simulink model "PowerFlow_SUSAN"  (R2022b)
settings: Solver=FixedStepAuto  StartTime=0.0  StopTime=10  FixedStep=0.02  RelTol=1e-3
libraries: Lib_EMTAT x193
(part 1 of 3)
settings Model: Creator=sbianco1  LastModifiedBy=sbianco1
settings SolverCC: AlgebraicLoopSolver=TrustRegion
settings DebuggingCC: UnconnectedInputMsg=warning  UnconnectedOutputMsg=warning  UnconnectedLineMsg=warning  SFMachineParentedDataDiag=warning
settings ModelReferenceCC: EnableRefExpFcnMdlSchedulingChecks=on
settings RTWCC: DLArmComputeVersion=19.05

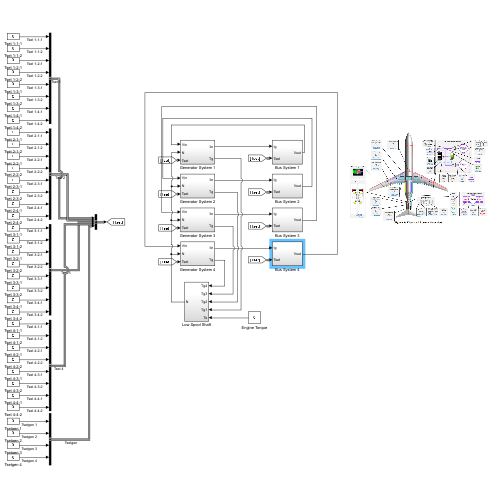
[thumbnail: Simulink's stored preview of the top-level diagram]
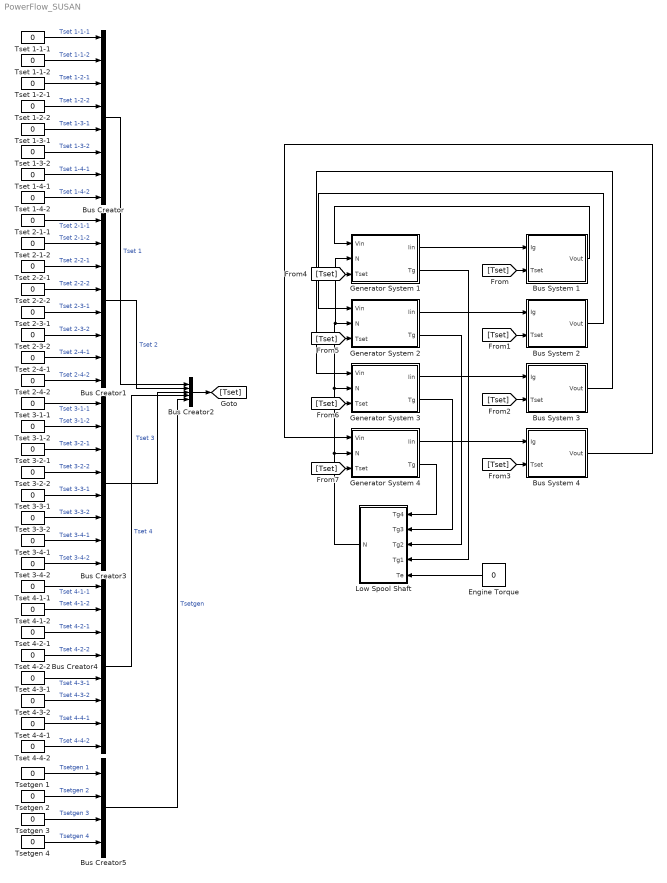
== system PowerFlow_SUSAN ==
  Bus Creator{,1,3..4} (4 alike) : BusCreator  Inputs=8
  Bus Creator2 : BusCreator  Inputs=5
  Bus Creator5 : BusCreator  Inputs=4
  Bus System 1 : Subsystem
  Bus System 2 : Subsystem
  Bus System 3 : Subsystem
  Bus System 4 : Subsystem
  Engine Torque : Constant  Value=0
  Generator System 1 : Subsystem
  Generator System 2 : Subsystem
  Generator System 3 : Subsystem
  Generator System 4 : Subsystem
  Low Spool Shaft : Subsystem
  Tset 1-1-1 : Constant  Value=0
  Tset 1-1-2 : Constant  Value=0
  Tset 1-2-1 : Constant  Value=0
  Tset 1-2-2 : Constant  Value=0
  Tset 1-3-1 : Constant  Value=0
  Tset 1-3-2 : Constant  Value=0
  Tset 1-4-1 : Constant  Value=0
  Tset 1-4-2 : Constant  Value=0
  Tset 2-1-1 : Constant  Value=0
  Tset 2-1-2 : Constant  Value=0
  Tset 2-2-1 : Constant  Value=0
  Tset 2-2-2 : Constant  Value=0
  Tset 2-3-1 : Constant  Value=0
  Tset 2-3-2 : Constant  Value=0
  Tset 2-4-1 : Constant  Value=0
  Tset 2-4-2 : Constant  Value=0
  Tset 3-1-1 : Constant  Value=0
  Tset 3-1-2 : Constant  Value=0
  Tset 3-2-1 : Constant  Value=0
  Tset 3-2-2 : Constant  Value=0
  Tset 3-3-1 : Constant  Value=0
  Tset 3-3-2 : Constant  Value=0
  Tset 3-4-1 : Constant  Value=0
  Tset 3-4-2 : Constant  Value=0
  Tset 4-1-1 : Constant  Value=0
  Tset 4-1-2 : Constant  Value=0
  Tset 4-2-1 : Constant  Value=0
  Tset 4-2-2 : Constant  Value=0
  Tset 4-3-1 : Constant  Value=0
  Tset 4-3-2 : Constant  Value=0
  Tset 4-4-1 : Constant  Value=0
  Tset 4-4-2 : Constant  Value=0
  Tsetgen {1..4} (4 alike) : Constant  Value=0
  wires:
  Engine Torque/1 -> Low Spool Shaft/5(Te)
  Generator System 1/2(Tg) -> Low Spool Shaft/4(Tg1)
  Generator System 2/2(Tg) -> Low Spool Shaft/3(Tg2)
  Generator System 3/2(Tg) -> Low Spool Shaft/2(Tg3)
  Generator System 4/2(Tg) -> Low Spool Shaft/1(Tg4)
  Low Spool Shaft/1(N) -> Generator System 4/2(N), Generator System 3/2(N), Generator System 2/2(N), Generator System 1/2(N)
  Generator System 1/1(Iin) -> Bus System 1/1(Ig)
  Bus System 1/1(Vout) -> Generator System 1/1(Vin)
  Generator System 2/1(Iin) -> Bus System 2/1(Ig)
  Generator System 3/1(Iin) -> Bus System 3/1(Ig)
  Generator System 4/1(Iin) -> Bus System 4/1(Ig)
  Bus System 2/1(Vout) -> Generator System 2/1(Vin)
  Bus System 3/1(Vout) -> Generator System 3/1(Vin)
  Bus System 4/1(Vout) -> Generator System 4/1(Vin)
  Tset 1-4-2/1 -> Bus Creator/8  "Tset 1-4-2"
  Tset 1-4-1/1 -> Bus Creator/7  "Tset 1-4-1"
  Tset 1-3-2/1 -> Bus Creator/6  "Tset 1-3-2"
  Tset 1-3-1/1 -> Bus Creator/5  "Tset 1-3-1"
  Tset 1-2-2/1 -> Bus Creator/4  "Tset 1-2-2"
  Tset 1-2-1/1 -> Bus Creator/3  "Tset 1-2-1"
  Tset 1-1-2/1 -> Bus Creator/2  "Tset 1-1-2"
  Tset 1-1-1/1 -> Bus Creator/1  "Tset 1-1-1"
  Bus Creator/1 -> Bus Creator2/1  "Tset 1"
  Bus Creator1/1 -> Bus Creator2/2  "Tset 2"
  Tset 2-1-1/1 -> Bus Creator1/1  "Tset 2-1-1"
  Tset 2-1-2/1 -> Bus Creator1/2  "Tset 2-1-2"
  Tset 2-2-1/1 -> Bus Creator1/3  "Tset 2-2-1"
  Tset 2-2-2/1 -> Bus Creator1/4  "Tset 2-2-2"
  Tset 2-3-1/1 -> Bus Creator1/5  "Tset 2-3-1"
  Tset 2-3-2/1 -> Bus Creator1/6  "Tset 2-3-2"
  Tset 2-4-1/1 -> Bus Creator1/7  "Tset 2-4-1"
  Tset 2-4-2/1 -> Bus Creator1/8  "Tset 2-4-2"
  Bus Creator2/1 -> [Tset]
  [Tset] -> Bus System 1/2(Tset)
  [Tset] -> Bus System 2/2(Tset)
  [Tset] -> Bus System 3/2(Tset)
  [Tset] -> Bus System 4/2(Tset)
  Tset 3-4-2/1 -> Bus Creator3/8  "Tset 3-4-2"
  Tset 3-4-1/1 -> Bus Creator3/7  "Tset 3-4-1"
  Tset 3-3-2/1 -> Bus Creator3/6  "Tset 3-3-2"
  Tset 3-3-1/1 -> Bus Creator3/5  "Tset 3-3-1"
  Tset 3-2-2/1 -> Bus Creator3/4  "Tset 3-2-2"
  Tset 3-2-1/1 -> Bus Creator3/3  "Tset 3-2-1"
  Tset 3-1-2/1 -> Bus Creator3/2  "Tset 3-1-2"
  Tset 3-1-1/1 -> Bus Creator3/1  "Tset 3-1-1"
  Bus Creator3/1 -> Bus Creator2/3  "Tset 3"
  Bus Creator4/1 -> Bus Creator2/4  "Tset 4"
  Tset 4-1-1/1 -> Bus Creator4/1  "Tset 4-1-1"
  Tset 4-1-2/1 -> Bus Creator4/2  "Tset 4-1-2"
  Tset 4-2-1/1 -> Bus Creator4/3  "Tset 4-2-1"
  Tset 4-2-2/1 -> Bus Creator4/4  "Tset 4-2-2"
  Tset 4-3-1/1 -> Bus Creator4/5  "Tset 4-3-1"
  Tset 4-3-2/1 -> Bus Creator4/6  "Tset 4-3-2"
  Tset 4-4-1/1 -> Bus Creator4/7  "Tset 4-4-1"
  Tset 4-4-2/1 -> Bus Creator4/8  "Tset 4-4-2"
  Tsetgen 1/1 -> Bus Creator5/1  "Tsetgen 1"
  Tsetgen 2/1 -> Bus Creator5/2  "Tsetgen 2"
  Tsetgen 3/1 -> Bus Creator5/3  "Tsetgen 3"
  Tsetgen 4/1 -> Bus Creator5/4  "Tsetgen 4"
  Bus Creator5/1 -> Bus Creator2/5  "Tsetgen"
  [Tset] -> Generator System 1/3(Tset)
  [Tset] -> Generator System 2/3(Tset)
  [Tset] -> Generator System 3/3(Tset)
  [Tset] -> Generator System 4/3(Tset)

== system PowerFlow_SUSAN/Bus System 1 ==
  Ig : Inport
  Tset : Inport  Port=2
  Bus Selector : BusSelector  OutputSignals=Tset 1.Tset 1-1-1,Tset 1.Tset 1-1-2  OutputAsBus=on
  Bus Selector1 : BusSelector  OutputSignals=Tset 1.Tset 1-2-1,Tset 1.Tset 1-2-2  OutputAsBus=on
  Bus Selector2 : BusSelector  OutputSignals=Tset 1.Tset 1-3-1,Tset 1.Tset 1-3-2  OutputAsBus=on
  Bus Selector3 : BusSelector  OutputSignals=Tset 1.Tset 1-4-1,Tset 1.Tset 1-4-2  OutputAsBus=on
  Current Distribution1 : Lib_EMTAT/Components/Power Flow/Current Distribution
      settings: SourceProductName=EMTAT
  Demux : Demux
  Mux : Mux
  Propulsor System 1 : Subsystem
  Propulsor System 2 : Subsystem
  Propulsor System 3 : Subsystem
  Propulsor System 4 : Subsystem
  Terminator : Terminator
  Terminator1 : Terminator
  Terminator2 : Terminator
  Vout : Outport
  wires:
  Propulsor System 3/2(Idmd) -> Mux/3
  Demux/1 -> Propulsor System 1/1(Iin)
  Demux/3 -> Propulsor System 3/1(Iin)
  Demux/4 -> Propulsor System 4/1(Iin)
  Propulsor System 3/1(Vout) -> Terminator1/1
  Propulsor System 2/2(Idmd) -> Mux/2
  Demux/2 -> Propulsor System 2/1(Iin)
  Propulsor System 4/1(Vout) -> Terminator2/1
  Propulsor System 2/1(Vout) -> Terminator/1
  Propulsor System 4/2(Idmd) -> Mux/4
  Propulsor System 1/2(Idmd) -> Mux/1
  Propulsor System 1/1(Vout) -> Vout/1
  Ig/1 -> Current Distribution1/1
  Tset/1 -> Bus Selector1/1, Bus Selector2/1, Bus Selector3/1, Bus Selector/1
  [Tset_1] -> Propulsor System 1/2(Tset)
  [Tset_2] -> Propulsor System 2/2(Tset)
  [Tset_3] -> Propulsor System 3/2(Tset)
  [Tset_4] -> Propulsor System 4/2(Tset)
  Bus Selector/1 -> [Tset_1]
  Bus Selector1/1 -> [Tset_2]
  Bus Selector2/1 -> [Tset_3]
  Bus Selector3/1 -> [Tset_4]
  Mux/1 -> Current Distribution1/2
  Current Distribution1/1 -> Demux/1

== system PowerFlow_SUSAN/Bus System 2 ==
  Ig : Inport
  Tset : Inport  Port=2
  Bus Selector : BusSelector  OutputSignals=Tset 2.Tset 2-1-1,Tset 2.Tset 2-1-2  OutputAsBus=on
  Bus Selector1 : BusSelector  OutputSignals=Tset 2.Tset 2-2-1,Tset 2.Tset 2-2-2  OutputAsBus=on
  Bus Selector2 : BusSelector  OutputSignals=Tset 2.Tset 2-3-1,Tset 2.Tset 2-3-2  OutputAsBus=on
  Bus Selector3 : BusSelector  OutputSignals=Tset 2.Tset 2-4-1,Tset 2.Tset 2-4-2  OutputAsBus=on
  Current Distribution1 : Lib_EMTAT/Components/Power Flow/Current Distribution
      settings: SourceProductName=EMTAT
  Demux : Demux
  Mux : Mux
  Propulsor System 1 : Subsystem
  Propulsor System 2 : Subsystem
  Propulsor System 3 : Subsystem
  Propulsor System 4 : Subsystem
  Terminator : Terminator
  Terminator1 : Terminator
  Terminator2 : Terminator
  Vout : Outport
  wires:
  Current Distribution1/1 -> Demux/1
  Mux/1 -> Current Distribution1/2
  Bus Selector3/1 -> [Tset_4]
  Bus Selector2/1 -> [Tset_3]
  Bus Selector1/1 -> [Tset_2]
  Bus Selector/1 -> [Tset_1]
  [Tset_4] -> Propulsor System 4/2(Tset)
  [Tset_3] -> Propulsor System 3/2(Tset)
  [Tset_2] -> Propulsor System 2/2(Tset)
  [Tset_1] -> Propulsor System 1/2(Tset)
  Tset/1 -> Bus Selector/1, Bus Selector3/1, Bus Selector2/1, Bus Selector1/1
  Ig/1 -> Current Distribution1/1
  Propulsor System 1/1(Vout) -> Vout/1
  Propulsor System 1/2(Idmd) -> Mux/1
  Propulsor System 4/2(Idmd) -> Mux/4
  Propulsor System 2/1(Vout) -> Terminator/1
  Propulsor System 4/1(Vout) -> Terminator2/1
  Demux/2 -> Propulsor System 2/1(Iin)
  Propulsor System 2/2(Idmd) -> Mux/2
  Propulsor System 3/1(Vout) -> Terminator1/1
  Demux/4 -> Propulsor System 4/1(Iin)
  Demux/3 -> Propulsor System 3/1(Iin)
  Demux/1 -> Propulsor System 1/1(Iin)
  Propulsor System 3/2(Idmd) -> Mux/3

== system PowerFlow_SUSAN/Bus System 3 ==
  Ig : Inport
  Tset : Inport  Port=2
  Bus Selector : BusSelector  OutputSignals=Tset 3.Tset 3-1-1,Tset 3.Tset 3-1-2  OutputAsBus=on
  Bus Selector1 : BusSelector  OutputSignals=Tset 3.Tset 3-2-1,Tset 3.Tset 3-2-2  OutputAsBus=on
  Bus Selector2 : BusSelector  OutputSignals=Tset 3.Tset 3-3-1,Tset 3.Tset 3-3-2  OutputAsBus=on
  Bus Selector3 : BusSelector  OutputSignals=Tset 3.Tset 3-4-1,Tset 3.Tset 3-4-2  OutputAsBus=on
  Current Distribution1 : Lib_EMTAT/Components/Power Flow/Current Distribution
      settings: SourceProductName=EMTAT
  Demux : Demux
  Mux : Mux
  Propulsor System 1 : Subsystem
  Propulsor System 2 : Subsystem
  Propulsor System 3 : Subsystem
  Propulsor System 4 : Subsystem
  Terminator : Terminator
  Terminator1 : Terminator
  Terminator2 : Terminator
  Vout : Outport
  wires:
  Propulsor System 3/2(Idmd) -> Mux/3
  Demux/1 -> Propulsor System 1/1(Iin)
  Demux/3 -> Propulsor System 3/1(Iin)
  Demux/4 -> Propulsor System 4/1(Iin)
  Propulsor System 3/1(Vout) -> Terminator1/1
  Propulsor System 2/2(Idmd) -> Mux/2
  Demux/2 -> Propulsor System 2/1(Iin)
  Propulsor System 4/1(Vout) -> Terminator2/1
  Propulsor System 2/1(Vout) -> Terminator/1
  Propulsor System 4/2(Idmd) -> Mux/4
  Propulsor System 1/2(Idmd) -> Mux/1
  Propulsor System 1/1(Vout) -> Vout/1
  Ig/1 -> Current Distribution1/1
  Tset/1 -> Bus Selector1/1, Bus Selector2/1, Bus Selector3/1, Bus Selector/1
  [Tset_1] -> Propulsor System 1/2(Tset)
  [Tset_2] -> Propulsor System 2/2(Tset)
  [Tset_3] -> Propulsor System 3/2(Tset)
  [Tset_4] -> Propulsor System 4/2(Tset)
  Bus Selector/1 -> [Tset_1]
  Bus Selector1/1 -> [Tset_2]
  Bus Selector2/1 -> [Tset_3]
  Bus Selector3/1 -> [Tset_4]
  Mux/1 -> Current Distribution1/2
  Current Distribution1/1 -> Demux/1

== system PowerFlow_SUSAN/Bus System 4 ==
  Ig : Inport
  Tset : Inport  Port=2
  Bus Selector : BusSelector  OutputSignals=Tset 4.Tset 4-1-1,Tset 4.Tset 4-1-2  OutputAsBus=on
  Bus Selector1 : BusSelector  OutputSignals=Tset 4.Tset 4-2-1,Tset 4.Tset 4-2-2  OutputAsBus=on
  Bus Selector2 : BusSelector  OutputSignals=Tset 4.Tset 4-3-1,Tset 4.Tset 4-3-2  OutputAsBus=on
  Bus Selector3 : BusSelector  OutputSignals=Tset 4.Tset 4-4-1,Tset 4.Tset 4-4-2  OutputAsBus=on
  Current Distribution1 : Lib_EMTAT/Components/Power Flow/Current Distribution
      settings: SourceProductName=EMTAT
  Demux : Demux
  Mux : Mux
  Propulsor System 1 : Subsystem
  Propulsor System 2 : Subsystem
  Propulsor System 3 : Subsystem
  Propulsor System 4 : Subsystem
  Terminator : Terminator
  Terminator1 : Terminator
  Terminator2 : Terminator
  Vout : Outport
  wires:
  Current Distribution1/1 -> Demux/1
  Mux/1 -> Current Distribution1/2
  Bus Selector3/1 -> [Tset_4]
  Bus Selector2/1 -> [Tset_3]
  Bus Selector1/1 -> [Tset_2]
  Bus Selector/1 -> [Tset_1]
  [Tset_4] -> Propulsor System 4/2(Tset)
  [Tset_3] -> Propulsor System 3/2(Tset)
  [Tset_2] -> Propulsor System 2/2(Tset)
  [Tset_1] -> Propulsor System 1/2(Tset)
  Tset/1 -> Bus Selector/1, Bus Selector3/1, Bus Selector2/1, Bus Selector1/1
  Ig/1 -> Current Distribution1/1
  Propulsor System 1/1(Vout) -> Vout/1
  Propulsor System 1/2(Idmd) -> Mux/1
  Propulsor System 4/2(Idmd) -> Mux/4
  Propulsor System 2/1(Vout) -> Terminator/1
  Propulsor System 4/1(Vout) -> Terminator2/1
  Demux/2 -> Propulsor System 2/1(Iin)
  Propulsor System 2/2(Idmd) -> Mux/2
  Propulsor System 3/1(Vout) -> Terminator1/1
  Demux/4 -> Propulsor System 4/1(Iin)
  Demux/3 -> Propulsor System 3/1(Iin)
  Demux/1 -> Propulsor System 1/1(Iin)
  Propulsor System 3/2(Idmd) -> Mux/3

== system PowerFlow_SUSAN/Generator System 1 ==
  Vin : Inport
  N : Inport  Port=2
  Tset : Inport  Port=3
  Bus Selector : BusSelector  OutputSignals=Tsetgen.Tsetgen 1
  Cable2 : Lib_EMTAT/Components/Power Flow/Cable  R=0.2
      settings: SourceProductName=EMTAT
  Constant{,1..4} (5 alike) : Constant  Value=0
  Inverter/Rectifier (Sink) : Lib_EMTAT/Components/Power Flow/DC-AC Inverter  X_C_VoltageInVec_M=[0 400]  Y_C_RMSCurrentOutVec_M=[0 300]  T_C_PowLossArray_M=[1000 1000; 1000 1000]  K_e=0.0503  FM=0  Plosslim=0
      settings: SourceProductName=EMTAT
  Motor/Generator (Sink)2 : Lib_EMTAT/Components/Power Flow/Three Phase Electric Machine (Sink)  X_C_SpeedVec_M=[0 100 1000 5000]  Y_C_TorqueVec_M=[0 10 100 150]  T_C_EffArray_M=0.99*ones(4,4)  FM=0
      settings: SourceProductName=EMTAT
  Terminator{1,9..10,14..16} (6 alike) : Terminator
  Unit Delay : UnitDelay  SampleTime=-1  HasFrameUpgradeWarning=on
  Iin : Outport
  Tg : Outport  Port=2
  wires:
  Unit Delay/1 -> Cable2/4
  Inverter/Rectifier (Sink)/2 -> Terminator15/1
  Motor/Generator (Sink)2/4 -> Inverter/Rectifier (Sink)/3
  Inverter/Rectifier (Sink)/4 -> Cable2/2
  Cable2/1 -> Inverter/Rectifier (Sink)/1
  Motor/Generator (Sink)2/1 -> Tg/1
  Tset/1 -> Bus Selector/1
  Cable2/5 -> Unit Delay/1
  [N_G] -> Inverter/Rectifier (Sink)/2
  Motor/Generator (Sink)2/2 -> Terminator16/1
  Inverter/Rectifier (Sink)/3 -> Terminator14/1
  Cable2/3 -> Terminator10/1
  Inverter/Rectifier (Sink)/1 -> Motor/Generator (Sink)2/1
  [N_G] -> Motor/Generator (Sink)2/2
  Cable2/2 -> Terminator9/1
  Vin/1 -> Cable2/1
  Cable2/4 -> Iin/1
  N/1 -> [N_G]
  Bus Selector/1 -> Motor/Generator (Sink)2/3  "<Tsetgen 1>"
  Constant/1 -> Inverter/Rectifier (Sink)/4
  Constant1/1 -> Cable2/3
  Constant2/1 -> Inverter/Rectifier (Sink)/5
  Constant3/1 -> Motor/Generator (Sink)2/4
  Constant4/1 -> Motor/Generator (Sink)2/5
  Motor/Generator (Sink)2/3 -> Terminator1/1

== system PowerFlow_SUSAN/Generator System 2 ==
  Vin : Inport
  N : Inport  Port=2
  Tset : Inport  Port=3
  Bus Selector : BusSelector  OutputSignals=Tsetgen.Tsetgen 1
  Cable2 : Lib_EMTAT/Components/Power Flow/Cable  R=0.2
      settings: SourceProductName=EMTAT
  Constant{,1..4} (5 alike) : Constant  Value=0
  Inverter/Rectifier (Sink) : Lib_EMTAT/Components/Power Flow/DC-AC Inverter  X_C_VoltageInVec_M=[0 400]  Y_C_RMSCurrentOutVec_M=[0 300]  T_C_PowLossArray_M=[1000 1000; 1000 1000]  K_e=0.0503  FM=0  Plosslim=0
      settings: SourceProductName=EMTAT
  Motor/Generator (Sink)2 : Lib_EMTAT/Components/Power Flow/Three Phase Electric Machine (Sink)  X_C_SpeedVec_M=[0 100 1000 5000]  Y_C_TorqueVec_M=[0 10 100 150]  T_C_EffArray_M=0.99*ones(4,4)  FM=0
      settings: SourceProductName=EMTAT
  Terminator{1,9..10,14..16} (6 alike) : Terminator
  Unit Delay : UnitDelay  SampleTime=-1  HasFrameUpgradeWarning=on
  Iin : Outport
  Tg : Outport  Port=2
  wires:
  Motor/Generator (Sink)2/3 -> Terminator1/1
  Constant4/1 -> Motor/Generator (Sink)2/5
  Constant3/1 -> Motor/Generator (Sink)2/4
  Constant2/1 -> Inverter/Rectifier (Sink)/5
  Constant1/1 -> Cable2/3
  Constant/1 -> Inverter/Rectifier (Sink)/4
  Bus Selector/1 -> Motor/Generator (Sink)2/3  "<Tsetgen 1>"
  N/1 -> [N_G]
  Cable2/4 -> Iin/1
  Vin/1 -> Cable2/1
  Cable2/2 -> Terminator9/1
  [N_G] -> Motor/Generator (Sink)2/2
  Inverter/Rectifier (Sink)/1 -> Motor/Generator (Sink)2/1
  Cable2/3 -> Terminator10/1
  Inverter/Rectifier (Sink)/3 -> Terminator14/1
  Motor/Generator (Sink)2/2 -> Terminator16/1
  [N_G] -> Inverter/Rectifier (Sink)/2
  Cable2/5 -> Unit Delay/1
  Tset/1 -> Bus Selector/1
  Motor/Generator (Sink)2/1 -> Tg/1
  Cable2/1 -> Inverter/Rectifier (Sink)/1
  Inverter/Rectifier (Sink)/4 -> Cable2/2
  Motor/Generator (Sink)2/4 -> Inverter/Rectifier (Sink)/3
  Inverter/Rectifier (Sink)/2 -> Terminator15/1
  Unit Delay/1 -> Cable2/4

== system PowerFlow_SUSAN/Generator System 3 ==
  Vin : Inport
  N : Inport  Port=2
  Tset : Inport  Port=3
  Bus Selector : BusSelector  OutputSignals=Tsetgen.Tsetgen 1
  Cable2 : Lib_EMTAT/Components/Power Flow/Cable  R=0.2
      settings: SourceProductName=EMTAT
  Constant{,1..4} (5 alike) : Constant  Value=0
  Inverter/Rectifier (Sink) : Lib_EMTAT/Components/Power Flow/DC-AC Inverter  X_C_VoltageInVec_M=[0 400]  Y_C_RMSCurrentOutVec_M=[0 300]  T_C_PowLossArray_M=[1000 1000; 1000 1000]  K_e=0.0503  FM=0  Plosslim=0
      settings: SourceProductName=EMTAT
  Motor/Generator (Sink)2 : Lib_EMTAT/Components/Power Flow/Three Phase Electric Machine (Sink)  X_C_SpeedVec_M=[0 100 1000 5000]  Y_C_TorqueVec_M=[0 10 100 150]  T_C_EffArray_M=0.99*ones(4,4)  FM=0
      settings: SourceProductName=EMTAT
  Terminator{1,9..10,14..16} (6 alike) : Terminator
  Unit Delay : UnitDelay  SampleTime=-1  HasFrameUpgradeWarning=on
  Iin : Outport
  Tg : Outport  Port=2
  wires:
  Unit Delay/1 -> Cable2/4
  Inverter/Rectifier (Sink)/2 -> Terminator15/1
  Motor/Generator (Sink)2/4 -> Inverter/Rectifier (Sink)/3
  Inverter/Rectifier (Sink)/4 -> Cable2/2
  Cable2/1 -> Inverter/Rectifier (Sink)/1
  Motor/Generator (Sink)2/1 -> Tg/1
  Tset/1 -> Bus Selector/1
  Cable2/5 -> Unit Delay/1
  [N_G] -> Inverter/Rectifier (Sink)/2
  Motor/Generator (Sink)2/2 -> Terminator16/1
  Inverter/Rectifier (Sink)/3 -> Terminator14/1
  Cable2/3 -> Terminator10/1
  Inverter/Rectifier (Sink)/1 -> Motor/Generator (Sink)2/1
  [N_G] -> Motor/Generator (Sink)2/2
  Cable2/2 -> Terminator9/1
  Vin/1 -> Cable2/1
  Cable2/4 -> Iin/1
  N/1 -> [N_G]
  Bus Selector/1 -> Motor/Generator (Sink)2/3  "<Tsetgen 1>"
  Constant/1 -> Inverter/Rectifier (Sink)/4
  Constant1/1 -> Cable2/3
  Constant2/1 -> Inverter/Rectifier (Sink)/5
  Constant3/1 -> Motor/Generator (Sink)2/4
  Constant4/1 -> Motor/Generator (Sink)2/5
  Motor/Generator (Sink)2/3 -> Terminator1/1

== system PowerFlow_SUSAN/Generator System 4 ==
  Vin : Inport
  N : Inport  Port=2
  Tset : Inport  Port=3
  Bus Selector : BusSelector  OutputSignals=Tsetgen.Tsetgen 1
  Cable2 : Lib_EMTAT/Components/Power Flow/Cable  R=0.2
      settings: SourceProductName=EMTAT
  Constant{,1..4} (5 alike) : Constant  Value=0
  Inverter/Rectifier (Sink) : Lib_EMTAT/Components/Power Flow/DC-AC Inverter  X_C_VoltageInVec_M=[0 400]  Y_C_RMSCurrentOutVec_M=[0 300]  T_C_PowLossArray_M=[1000 1000; 1000 1000]  K_e=0.0503  FM=0  Plosslim=0
      settings: SourceProductName=EMTAT
  Motor/Generator (Sink)2 : Lib_EMTAT/Components/Power Flow/Three Phase Electric Machine (Sink)  X_C_SpeedVec_M=[0 100 1000 5000]  Y_C_TorqueVec_M=[0 10 100 150]  T_C_EffArray_M=0.99*ones(4,4)  FM=0
      settings: SourceProductName=EMTAT
  Terminator{1,9..10,14..16} (6 alike) : Terminator
  Unit Delay : UnitDelay  SampleTime=-1  HasFrameUpgradeWarning=on
  Iin : Outport
  Tg : Outport  Port=2
  wires:
  Motor/Generator (Sink)2/3 -> Terminator1/1
  Constant4/1 -> Motor/Generator (Sink)2/5
  Constant3/1 -> Motor/Generator (Sink)2/4
  Constant2/1 -> Inverter/Rectifier (Sink)/5
  Constant1/1 -> Cable2/3
  Constant/1 -> Inverter/Rectifier (Sink)/4
  Bus Selector/1 -> Motor/Generator (Sink)2/3  "<Tsetgen 1>"
  N/1 -> [N_G]
  Cable2/4 -> Iin/1
  Vin/1 -> Cable2/1
  Cable2/2 -> Terminator9/1
  [N_G] -> Motor/Generator (Sink)2/2
  Inverter/Rectifier (Sink)/1 -> Motor/Generator (Sink)2/1
  Cable2/3 -> Terminator10/1
  Inverter/Rectifier (Sink)/3 -> Terminator14/1
  Motor/Generator (Sink)2/2 -> Terminator16/1
  [N_G] -> Inverter/Rectifier (Sink)/2
  Cable2/5 -> Unit Delay/1
  Tset/1 -> Bus Selector/1
  Motor/Generator (Sink)2/1 -> Tg/1
  Cable2/1 -> Inverter/Rectifier (Sink)/1
  Inverter/Rectifier (Sink)/4 -> Cable2/2
  Motor/Generator (Sink)2/4 -> Inverter/Rectifier (Sink)/3
  Inverter/Rectifier (Sink)/2 -> Terminator15/1
  Unit Delay/1 -> Cable2/4

== system PowerFlow_SUSAN/Low Spool Shaft ==
  Tg4 : Inport
  Tg3 : Inport  Port=2
  Tg2 : Inport  Port=3
  Tg1 : Inport  Port=4
  Te : Inport  Port=5
  Constant : Constant  Value=0
  Integrator : Integrator  InitialCondition=5000
  Mechanical Shaft3 : Lib_EMTAT/Components/Power Flow/Mechanical Shaft  J=0.01  B=0.001
      settings: SourceProductName=EMTAT
  Mux1 : Mux  Inputs=5
  Terminator5 : Terminator
  Terminator7 : Terminator
  N : Outport
  wires:
  Mux1/1 -> Mechanical Shaft3/1
  Integrator/1 -> Mechanical Shaft3/3, N/1
  Tg1/1 -> Mux1/1
  Tg4/1 -> Mux1/4
  Tg3/1 -> Mux1/3
  Tg2/1 -> Mux1/2
  Te/1 -> Mux1/5
  Mechanical Shaft3/1 -> Terminator5/1
  Mechanical Shaft3/2 -> Terminator7/1
  Mechanical Shaft3/3 -> Integrator/1
  Constant/1 -> Mechanical Shaft3/2

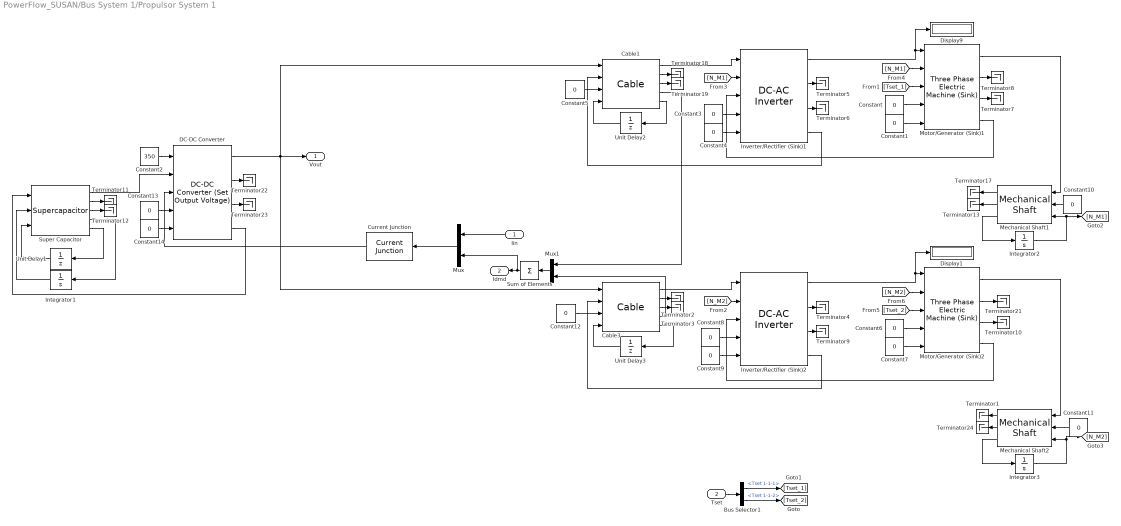
== system PowerFlow_SUSAN/Bus System 1/Propulsor System 1 ==
  Iin : Inport
  Tset : Inport  Port=2
  Bus Selector1 : BusSelector  OutputSignals=Tset 1-1-1,Tset 1-1-2
  Cable1 : Lib_EMTAT/Components/Power Flow/Cable  R=0.2
      settings: SourceProductName=EMTAT
  Cable3 : Lib_EMTAT/Components/Power Flow/Cable  R=0.2
      settings: SourceProductName=EMTAT
  Constant{,1,3..14} (14 alike) : Constant  Value=0
  Constant2 : Constant  Value=350
  Current Junction : Lib_EMTAT/Components/Power Flow/Current Junction  Nb=1
      settings: SourceProductName=EMTAT
      settings: AttributesFormatString=|
      | Current Junction
      | Version: %<LibraryVersion>
  DC-DC Converter : Lib_EMTAT/Components/Power Flow/DC-DC Converter (Set Output Voltage)  X_Vin_VoltageVec_M=[0 100 1000 5000]  Y_Iout_CurrentVec_M=[0 10 100 150]  T_C_PlossArray_M=0.98*ones(4,4)  FM=0  Plosslim=0
      settings: SourceProductName=EMTAT
  Display1 : Display
  Display9 : Display
  Integrator1 : Integrator  InitialCondition=150
  Integrator2 : Integrator  InitialCondition=2000
  Integrator3 : Integrator  InitialCondition=2000
  Inverter/Rectifier (Sink)1 : Lib_EMTAT/Components/Power Flow/DC-AC Inverter  X_C_VoltageInVec_M=[0 400]  Y_C_RMSCurrentOutVec_M=[0 300]  T_C_PowLossArray_M=[1000 1000;1000 1000]  K_e=0.0503  FM=0  Plosslim=0
      settings: SourceProductName=EMTAT
  Inverter/Rectifier (Sink)2 : Lib_EMTAT/Components/Power Flow/DC-AC Inverter  X_C_VoltageInVec_M=[0 400]  Y_C_RMSCurrentOutVec_M=[0 300]  T_C_PowLossArray_M=[1000 1000;1000 1000]  K_e=0.0503  FM=0  Plosslim=0
      settings: SourceProductName=EMTAT
  Mechanical Shaft1 : Lib_EMTAT/Components/Power Flow/Mechanical Shaft  J=0.01  B=0.001
      settings: SourceProductName=EMTAT
  Mechanical Shaft2 : Lib_EMTAT/Components/Power Flow/Mechanical Shaft  J=0.01  B=0.001
      settings: SourceProductName=EMTAT
  Motor/Generator (Sink)1 : Lib_EMTAT/Components/Power Flow/Three Phase Electric Machine (Sink)  X_C_SpeedVec_M=[0 100 1000 5000]  Y_C_TorqueVec_M=[0 10 100 150]  T_C_EffArray_M=0.99*ones(4,4)  FM=0
      settings: SourceProductName=EMTAT
  Motor/Generator (Sink)2 : Lib_EMTAT/Components/Power Flow/Three Phase Electric Machine (Sink)  X_C_SpeedVec_M=[0 100 1000 5000]  Y_C_TorqueVec_M=[0 10 100 150]  T_C_EffArray_M=0.99*ones(4,4)  FM=0
      settings: SourceProductName=EMTAT
  Mux : Mux  Inputs=2
  Mux1 : Mux  Inputs=2
  Sum of Elements : Sum  Inputs=+
  Super Capacitor : Lib_EMTAT/Components/Power Flow/Supercapacitor  C=130  ESR=0.02  TSE=0  BlkNm=double(gcb)
      settings: SourceProductName=EMTAT
  Terminator{1..13,17..19,21..24} (20 alike) : Terminator
  Unit Delay1 : UnitDelay  SampleTime=-1  HasFrameUpgradeWarning=on
  Unit Delay2 : UnitDelay  SampleTime=-1  HasFrameUpgradeWarning=on
  Unit Delay3 : UnitDelay  SampleTime=-1  HasFrameUpgradeWarning=on
  Vout : Outport
  Idmd : Outport  Port=2
  wires:
  Iin/1 -> Mux/1
  Mechanical Shaft2/3 -> Integrator3/1
  [Tset_1] -> Motor/Generator (Sink)1/3
  DC-DC Converter/1 -> Cable3/1, Vout/1, Cable1/1
  Motor/Generator (Sink)1/4 -> Inverter/Rectifier (Sink)1/3
  Super Capacitor/4 -> Integrator1/1
  Super Capacitor/1 -> DC-DC Converter/2
  [N_M1] -> Motor/Generator (Sink)1/2
  Mechanical Shaft1/2 -> Terminator13/1
  Unit Delay2/1 -> Cable1/4
  Cable3/2 -> Terminator2/1
  DC-DC Converter/4 -> Super Capacitor/1
  Current Junction/1 -> DC-DC Converter/3
  Mux/1 -> Current Junction/1
  Integrator2/1 -> [N_M1], Mechanical Shaft1/3
  Cable1/1 -> Inverter/Rectifier (Sink)1/1
  [N_M1] -> Inverter/Rectifier (Sink)1/2
  Cable3/5 -> Unit Delay3/1
  Inverter/Rectifier (Sink)1/1 -> Motor/Generator (Sink)1/1, Display9/1
  Super Capacitor/2 -> Terminator11/1
  Cable3/4 -> Mux1/2
  Integrator3/1 -> [N_M2], Mechanical Shaft2/3
  Cable1/3 -> Terminator19/1
  Unit Delay3/1 -> Cable3/4
  Inverter/Rectifier (Sink)1/4 -> Cable1/2
  Integrator1/1 -> Super Capacitor/2
  Cable1/5 -> Unit Delay2/1
  Inverter/Rectifier (Sink)1/3 -> Terminator6/1
  Super Capacitor/5 -> Unit Delay1/1
  Unit Delay1/1 -> Super Capacitor/3
  Cable1/4 -> Mux1/1
  Constant2/1 -> DC-DC Converter/1
  Motor/Generator (Sink)1/2 -> Terminator8/1
  Cable3/3 -> Terminator3/1
  Motor/Generator (Sink)2/1 -> Mechanical Shaft2/1
  Cable1/2 -> Terminator18/1
  Super Capacitor/3 -> Terminator12/1
  Motor/Generator (Sink)2/2 -> Terminator21/1
  Mechanical Shaft1/1 -> Terminator17/1
  DC-DC Converter/2 -> Terminator22/1
  DC-DC Converter/3 -> Terminator23/1
  Inverter/Rectifier (Sink)1/2 -> Terminator5/1
  Motor/Generator (Sink)1/1 -> Mechanical Shaft1/1
  Mux1/1 -> Sum of Elements/1
  Sum of Elements/1 -> Mux/2, Idmd/1
  Bus Selector1/1 -> [Tset_1]  "<Tset 1-1-1>"
  Bus Selector1/2 -> [Tset_2]  "<Tset 1-1-2>"
  Tset/1 -> Bus Selector1/1
  Constant/1 -> Motor/Generator (Sink)1/4
  Constant1/1 -> Motor/Generator (Sink)1/5
  Motor/Generator (Sink)1/3 -> Terminator7/1
  Constant3/1 -> Inverter/Rectifier (Sink)1/4
  Constant4/1 -> Inverter/Rectifier (Sink)1/5
  Constant5/1 -> Cable1/3
  Constant9/1 -> Inverter/Rectifier (Sink)2/5
  Inverter/Rectifier (Sink)2/2 -> Terminator4/1
  Constant7/1 -> Motor/Generator (Sink)2/5
  [N_M2] -> Inverter/Rectifier (Sink)2/2
  Inverter/Rectifier (Sink)2/3 -> Terminator9/1
  [Tset_2] -> Motor/Generator (Sink)2/3
  Inverter/Rectifier (Sink)2/4 -> Cable3/2
  Constant6/1 -> Motor/Generator (Sink)2/4
  Motor/Generator (Sink)2/4 -> Inverter/Rectifier (Sink)2/3
  Cable3/1 -> Inverter/Rectifier (Sink)2/1
  [N_M2] -> Motor/Generator (Sink)2/2
  Inverter/Rectifier (Sink)2/1 -> Motor/Generator (Sink)2/1, Display1/1
  Constant8/1 -> Inverter/Rectifier (Sink)2/4
  Motor/Generator (Sink)2/3 -> Terminator10/1
  Mechanical Shaft1/3 -> Integrator2/1
  Constant10/1 -> Mechanical Shaft1/2
  Constant11/1 -> Mechanical Shaft2/2
  Mechanical Shaft2/1 -> Terminator1/1
  Mechanical Shaft2/2 -> Terminator24/1
  Constant12/1 -> Cable3/3
  Constant13/1 -> DC-DC Converter/4
  Constant14/1 -> DC-DC Converter/5

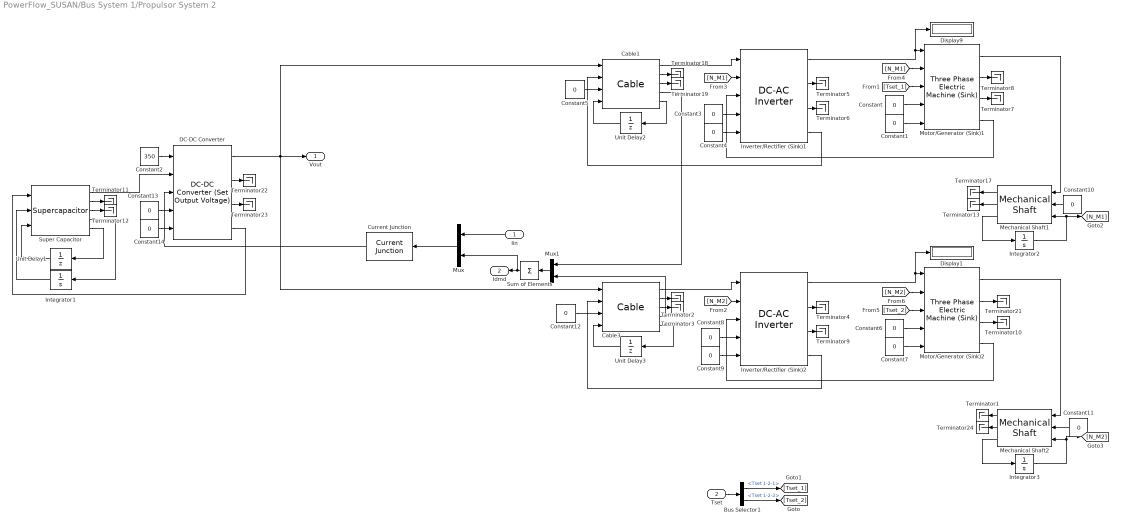
== system PowerFlow_SUSAN/Bus System 1/Propulsor System 2 ==
  Iin : Inport
  Tset : Inport  Port=2
  Bus Selector1 : BusSelector  OutputSignals=Tset 1-2-1,Tset 1-2-2
  Cable1 : Lib_EMTAT/Components/Power Flow/Cable  R=0.2
      settings: SourceProductName=EMTAT
  Cable3 : Lib_EMTAT/Components/Power Flow/Cable  R=0.2
      settings: SourceProductName=EMTAT
  Constant{,1,3..14} (14 alike) : Constant  Value=0
  Constant2 : Constant  Value=350
  Current Junction : Lib_EMTAT/Components/Power Flow/Current Junction  Nb=1
      settings: SourceProductName=EMTAT
      settings: AttributesFormatString=|
      | Current Junction
      | Version: %<LibraryVersion>
  DC-DC Converter : Lib_EMTAT/Components/Power Flow/DC-DC Converter (Set Output Voltage)  X_Vin_VoltageVec_M=[0 100 1000 5000]  Y_Iout_CurrentVec_M=[0 10 100 150]  T_C_PlossArray_M=0.98*ones(4,4)  FM=0  Plosslim=0
      settings: SourceProductName=EMTAT
  Display1 : Display
  Display9 : Display
  Integrator1 : Integrator  InitialCondition=150
  Integrator2 : Integrator  InitialCondition=2000
  Integrator3 : Integrator  InitialCondition=2000
  Inverter/Rectifier (Sink)1 : Lib_EMTAT/Components/Power Flow/DC-AC Inverter  X_C_VoltageInVec_M=[0 400]  Y_C_RMSCurrentOutVec_M=[0 300]  T_C_PowLossArray_M=[1000 1000;1000 1000]  K_e=0.0503  FM=0  Plosslim=0
      settings: SourceProductName=EMTAT
  Inverter/Rectifier (Sink)2 : Lib_EMTAT/Components/Power Flow/DC-AC Inverter  X_C_VoltageInVec_M=[0 400]  Y_C_RMSCurrentOutVec_M=[0 300]  T_C_PowLossArray_M=[1000 1000;1000 1000]  K_e=0.0503  FM=0  Plosslim=0
      settings: SourceProductName=EMTAT
  Mechanical Shaft1 : Lib_EMTAT/Components/Power Flow/Mechanical Shaft  J=0.01  B=0.001
      settings: SourceProductName=EMTAT
  Mechanical Shaft2 : Lib_EMTAT/Components/Power Flow/Mechanical Shaft  J=0.01  B=0.001
      settings: SourceProductName=EMTAT
  Motor/Generator (Sink)1 : Lib_EMTAT/Components/Power Flow/Three Phase Electric Machine (Sink)  X_C_SpeedVec_M=[0 100 1000 5000]  Y_C_TorqueVec_M=[0 10 100 150]  T_C_EffArray_M=0.99*ones(4,4)  FM=0
      settings: SourceProductName=EMTAT
  Motor/Generator (Sink)2 : Lib_EMTAT/Components/Power Flow/Three Phase Electric Machine (Sink)  X_C_SpeedVec_M=[0 100 1000 5000]  Y_C_TorqueVec_M=[0 10 100 150]  T_C_EffArray_M=0.99*ones(4,4)  FM=0
      settings: SourceProductName=EMTAT
  Mux : Mux  Inputs=2
  Mux1 : Mux  Inputs=2
  Sum of Elements : Sum  Inputs=+
  Super Capacitor : Lib_EMTAT/Components/Power Flow/Supercapacitor  C=130  ESR=0.02  TSE=0  BlkNm=double(gcb)
      settings: SourceProductName=EMTAT
  Terminator{1..13,17..19,21..24} (20 alike) : Terminator
  Unit Delay1 : UnitDelay  SampleTime=-1  HasFrameUpgradeWarning=on
  Unit Delay2 : UnitDelay  SampleTime=-1  HasFrameUpgradeWarning=on
  Unit Delay3 : UnitDelay  SampleTime=-1  HasFrameUpgradeWarning=on
  Vout : Outport
  Idmd : Outport  Port=2
  wires:
  Constant14/1 -> DC-DC Converter/5
  Constant13/1 -> DC-DC Converter/4
  Constant12/1 -> Cable3/3
  Mechanical Shaft2/2 -> Terminator24/1
  Mechanical Shaft2/1 -> Terminator1/1
  Constant11/1 -> Mechanical Shaft2/2
  Constant10/1 -> Mechanical Shaft1/2
  Mechanical Shaft1/3 -> Integrator2/1
  Motor/Generator (Sink)2/3 -> Terminator10/1
  Constant8/1 -> Inverter/Rectifier (Sink)2/4
  Inverter/Rectifier (Sink)2/1 -> Display1/1, Motor/Generator (Sink)2/1
  [N_M2] -> Motor/Generator (Sink)2/2
  Cable3/1 -> Inverter/Rectifier (Sink)2/1
  Motor/Generator (Sink)2/4 -> Inverter/Rectifier (Sink)2/3
  Constant6/1 -> Motor/Generator (Sink)2/4
  Inverter/Rectifier (Sink)2/4 -> Cable3/2
  [Tset_2] -> Motor/Generator (Sink)2/3
  Inverter/Rectifier (Sink)2/3 -> Terminator9/1
  [N_M2] -> Inverter/Rectifier (Sink)2/2
  Constant7/1 -> Motor/Generator (Sink)2/5
  Inverter/Rectifier (Sink)2/2 -> Terminator4/1
  Constant9/1 -> Inverter/Rectifier (Sink)2/5
  Constant5/1 -> Cable1/3
  Constant4/1 -> Inverter/Rectifier (Sink)1/5
  Constant3/1 -> Inverter/Rectifier (Sink)1/4
  Motor/Generator (Sink)1/3 -> Terminator7/1
  Constant1/1 -> Motor/Generator (Sink)1/5
  Constant/1 -> Motor/Generator (Sink)1/4
  Tset/1 -> Bus Selector1/1
  Bus Selector1/2 -> [Tset_2]  "<Tset 1-2-2>"
  Bus Selector1/1 -> [Tset_1]  "<Tset 1-2-1>"
  Sum of Elements/1 -> Idmd/1, Mux/2
  Mux1/1 -> Sum of Elements/1
  Motor/Generator (Sink)1/1 -> Mechanical Shaft1/1
  Inverter/Rectifier (Sink)1/2 -> Terminator5/1
  DC-DC Converter/3 -> Terminator23/1
  DC-DC Converter/2 -> Terminator22/1
  Mechanical Shaft1/1 -> Terminator17/1
  Motor/Generator (Sink)2/2 -> Terminator21/1
  Super Capacitor/3 -> Terminator12/1
  Cable1/2 -> Terminator18/1
  Motor/Generator (Sink)2/1 -> Mechanical Shaft2/1
  Cable3/3 -> Terminator3/1
  Motor/Generator (Sink)1/2 -> Terminator8/1
  Constant2/1 -> DC-DC Converter/1
  Cable1/4 -> Mux1/1
  Unit Delay1/1 -> Super Capacitor/3
  Super Capacitor/5 -> Unit Delay1/1
  Inverter/Rectifier (Sink)1/3 -> Terminator6/1
  Cable1/5 -> Unit Delay2/1
  Integrator1/1 -> Super Capacitor/2
  Inverter/Rectifier (Sink)1/4 -> Cable1/2
  Unit Delay3/1 -> Cable3/4
  Cable1/3 -> Terminator19/1
  Integrator3/1 -> Mechanical Shaft2/3, [N_M2]
  Cable3/4 -> Mux1/2
  Super Capacitor/2 -> Terminator11/1
  Inverter/Rectifier (Sink)1/1 -> Display9/1, Motor/Generator (Sink)1/1
  Cable3/5 -> Unit Delay3/1
  [N_M1] -> Inverter/Rectifier (Sink)1/2
  Cable1/1 -> Inverter/Rectifier (Sink)1/1
  Integrator2/1 -> Mechanical Shaft1/3, [N_M1]
  Mux/1 -> Current Junction/1
  Current Junction/1 -> DC-DC Converter/3
  DC-DC Converter/4 -> Super Capacitor/1
  Cable3/2 -> Terminator2/1
  Unit Delay2/1 -> Cable1/4
  Mechanical Shaft1/2 -> Terminator13/1
  [N_M1] -> Motor/Generator (Sink)1/2
  Super Capacitor/1 -> DC-DC Converter/2
  Super Capacitor/4 -> Integrator1/1
  Motor/Generator (Sink)1/4 -> Inverter/Rectifier (Sink)1/3
  DC-DC Converter/1 -> Cable1/1, Vout/1, Cable3/1
  [Tset_1] -> Motor/Generator (Sink)1/3
  Mechanical Shaft2/3 -> Integrator3/1
  Iin/1 -> Mux/1

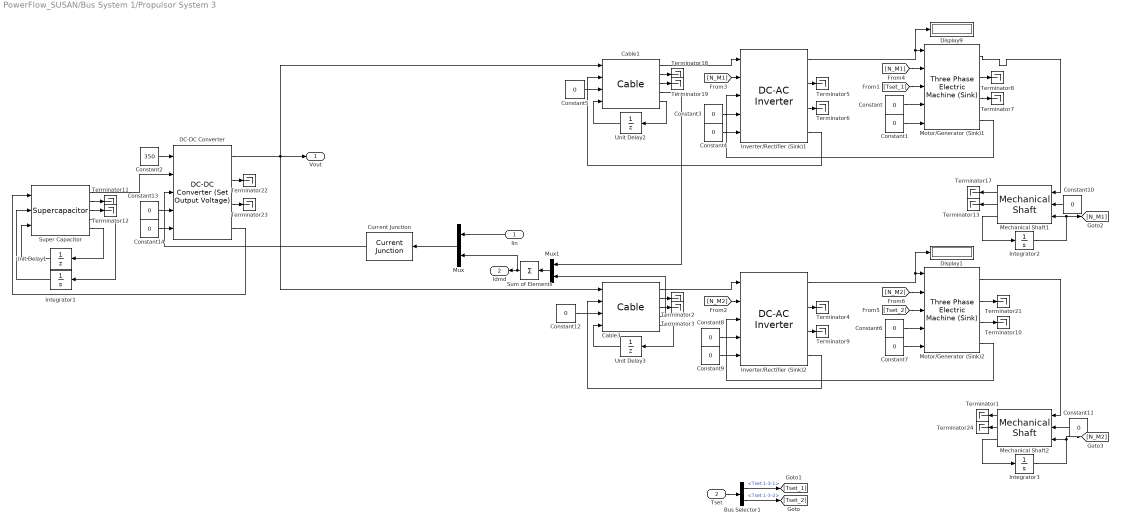
== system PowerFlow_SUSAN/Bus System 1/Propulsor System 3 ==
  Iin : Inport
  Tset : Inport  Port=2
  Bus Selector1 : BusSelector  OutputSignals=Tset 1-3-1,Tset 1-3-2
  Cable1 : Lib_EMTAT/Components/Power Flow/Cable  R=0.2
      settings: SourceProductName=EMTAT
  Cable3 : Lib_EMTAT/Components/Power Flow/Cable  R=0.2
      settings: SourceProductName=EMTAT
  Constant{,1,3..14} (14 alike) : Constant  Value=0
  Constant2 : Constant  Value=350
  Current Junction : Lib_EMTAT/Components/Power Flow/Current Junction  Nb=1
      settings: SourceProductName=EMTAT
      settings: AttributesFormatString=|
      | Current Junction
      | Version: %<LibraryVersion>
  DC-DC Converter : Lib_EMTAT/Components/Power Flow/DC-DC Converter (Set Output Voltage)  X_Vin_VoltageVec_M=[0 100 1000 5000]  Y_Iout_CurrentVec_M=[0 10 100 150]  T_C_PlossArray_M=0.98*ones(4,4)  FM=0  Plosslim=0
      settings: SourceProductName=EMTAT
  Display1 : Display
  Display9 : Display
  Integrator1 : Integrator  InitialCondition=150
  Integrator2 : Integrator  InitialCondition=2000
  Integrator3 : Integrator  InitialCondition=2000
  Inverter/Rectifier (Sink)1 : Lib_EMTAT/Components/Power Flow/DC-AC Inverter  X_C_VoltageInVec_M=[0 400]  Y_C_RMSCurrentOutVec_M=[0 300]  T_C_PowLossArray_M=[1000 1000;1000 1000]  K_e=0.0503  FM=0  Plosslim=0
      settings: SourceProductName=EMTAT
  Inverter/Rectifier (Sink)2 : Lib_EMTAT/Components/Power Flow/DC-AC Inverter  X_C_VoltageInVec_M=[0 400]  Y_C_RMSCurrentOutVec_M=[0 300]  T_C_PowLossArray_M=[1000 1000;1000 1000]  K_e=0.0503  FM=0  Plosslim=0
      settings: SourceProductName=EMTAT
  Mechanical Shaft1 : Lib_EMTAT/Components/Power Flow/Mechanical Shaft  J=0.01  B=0.001
      settings: SourceProductName=EMTAT
  Mechanical Shaft2 : Lib_EMTAT/Components/Power Flow/Mechanical Shaft  J=0.01  B=0.001
      settings: SourceProductName=EMTAT
  Motor/Generator (Sink)1 : Lib_EMTAT/Components/Power Flow/Three Phase Electric Machine (Sink)  X_C_SpeedVec_M=[0 100 1000 5000]  Y_C_TorqueVec_M=[0 10 100 150]  T_C_EffArray_M=0.99*ones(4,4)  FM=0
      settings: SourceProductName=EMTAT
  Motor/Generator (Sink)2 : Lib_EMTAT/Components/Power Flow/Three Phase Electric Machine (Sink)  X_C_SpeedVec_M=[0 100 1000 5000]  Y_C_TorqueVec_M=[0 10 100 150]  T_C_EffArray_M=0.99*ones(4,4)  FM=0
      settings: SourceProductName=EMTAT
  Mux : Mux  Inputs=2
  Mux1 : Mux  Inputs=2
  Sum of Elements : Sum  Inputs=+
  Super Capacitor : Lib_EMTAT/Components/Power Flow/Supercapacitor  C=130  ESR=0.02  TSE=0  BlkNm=double(gcb)
      settings: SourceProductName=EMTAT
  Terminator{1..13,17..19,21..24} (20 alike) : Terminator
  Unit Delay1 : UnitDelay  SampleTime=-1  HasFrameUpgradeWarning=on
  Unit Delay2 : UnitDelay  SampleTime=-1  HasFrameUpgradeWarning=on
  Unit Delay3 : UnitDelay  SampleTime=-1  HasFrameUpgradeWarning=on
  Vout : Outport
  Idmd : Outport  Port=2
  wires:
  Iin/1 -> Mux/1
  Mechanical Shaft2/3 -> Integrator3/1
  [Tset_1] -> Motor/Generator (Sink)1/3
  DC-DC Converter/1 -> Cable3/1, Vout/1, Cable1/1
  Motor/Generator (Sink)1/4 -> Inverter/Rectifier (Sink)1/3
  Super Capacitor/4 -> Integrator1/1
  Super Capacitor/1 -> DC-DC Converter/2
  [N_M1] -> Motor/Generator (Sink)1/2
  Mechanical Shaft1/2 -> Terminator13/1
  Unit Delay2/1 -> Cable1/4
  Cable3/2 -> Terminator2/1
  DC-DC Converter/4 -> Super Capacitor/1
  Current Junction/1 -> DC-DC Converter/3
  Mux/1 -> Current Junction/1
  Integrator2/1 -> [N_M1], Mechanical Shaft1/3
  Cable1/1 -> Inverter/Rectifier (Sink)1/1
  [N_M1] -> Inverter/Rectifier (Sink)1/2
  Cable3/5 -> Unit Delay3/1
  Inverter/Rectifier (Sink)1/1 -> Motor/Generator (Sink)1/1, Display9/1
  Super Capacitor/2 -> Terminator11/1
  Cable3/4 -> Mux1/2
  Integrator3/1 -> [N_M2], Mechanical Shaft2/3
  Cable1/3 -> Terminator19/1
  Unit Delay3/1 -> Cable3/4
  Inverter/Rectifier (Sink)1/4 -> Cable1/2
  Integrator1/1 -> Super Capacitor/2
  Cable1/5 -> Unit Delay2/1
  Inverter/Rectifier (Sink)1/3 -> Terminator6/1
  Super Capacitor/5 -> Unit Delay1/1
  Unit Delay1/1 -> Super Capacitor/3
  Cable1/4 -> Mux1/1
  Constant2/1 -> DC-DC Converter/1
  Motor/Generator (Sink)1/2 -> Terminator8/1
  Cable3/3 -> Terminator3/1
  Motor/Generator (Sink)2/1 -> Mechanical Shaft2/1
  Cable1/2 -> Terminator18/1
  Super Capacitor/3 -> Terminator12/1
  Motor/Generator (Sink)2/2 -> Terminator21/1
  Mechanical Shaft1/1 -> Terminator17/1
  DC-DC Converter/2 -> Terminator22/1
  DC-DC Converter/3 -> Terminator23/1
  Inverter/Rectifier (Sink)1/2 -> Terminator5/1
  Motor/Generator (Sink)1/1 -> Mechanical Shaft1/1
  Mux1/1 -> Sum of Elements/1
  Sum of Elements/1 -> Mux/2, Idmd/1
  Bus Selector1/1 -> [Tset_1]  "<Tset 1-3-1>"
  Bus Selector1/2 -> [Tset_2]  "<Tset 1-3-2>"
  Tset/1 -> Bus Selector1/1
  Constant/1 -> Motor/Generator (Sink)1/4
  Constant1/1 -> Motor/Generator (Sink)1/5
  Motor/Generator (Sink)1/3 -> Terminator7/1
  Constant3/1 -> Inverter/Rectifier (Sink)1/4
  Constant4/1 -> Inverter/Rectifier (Sink)1/5
  Constant5/1 -> Cable1/3
  Constant9/1 -> Inverter/Rectifier (Sink)2/5
  Inverter/Rectifier (Sink)2/2 -> Terminator4/1
  Constant7/1 -> Motor/Generator (Sink)2/5
  [N_M2] -> Inverter/Rectifier (Sink)2/2
  Inverter/Rectifier (Sink)2/3 -> Terminator9/1
  [Tset_2] -> Motor/Generator (Sink)2/3
  Inverter/Rectifier (Sink)2/4 -> Cable3/2
  Constant6/1 -> Motor/Generator (Sink)2/4
  Motor/Generator (Sink)2/4 -> Inverter/Rectifier (Sink)2/3
  Cable3/1 -> Inverter/Rectifier (Sink)2/1
  [N_M2] -> Motor/Generator (Sink)2/2
  Inverter/Rectifier (Sink)2/1 -> Motor/Generator (Sink)2/1, Display1/1
  Constant8/1 -> Inverter/Rectifier (Sink)2/4
  Motor/Generator (Sink)2/3 -> Terminator10/1
  Mechanical Shaft1/3 -> Integrator2/1
  Constant10/1 -> Mechanical Shaft1/2
  Constant11/1 -> Mechanical Shaft2/2
  Mechanical Shaft2/1 -> Terminator1/1
  Mechanical Shaft2/2 -> Terminator24/1
  Constant12/1 -> Cable3/3
  Constant13/1 -> DC-DC Converter/4
  Constant14/1 -> DC-DC Converter/5

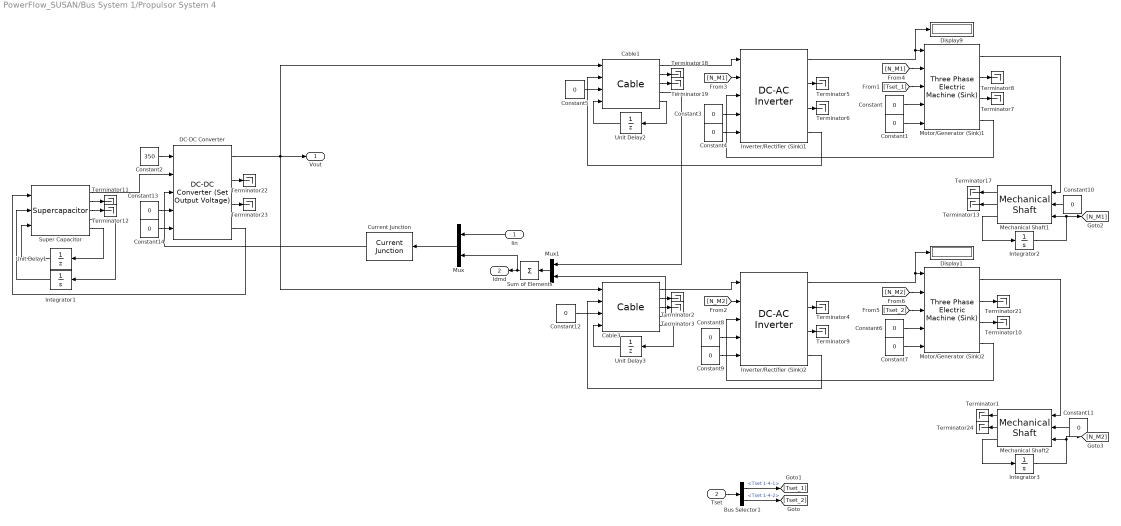
== system PowerFlow_SUSAN/Bus System 1/Propulsor System 4 ==
  Iin : Inport
  Tset : Inport  Port=2
  Bus Selector1 : BusSelector  OutputSignals=Tset 1-4-1,Tset 1-4-2
  Cable1 : Lib_EMTAT/Components/Power Flow/Cable  R=0.2
      settings: SourceProductName=EMTAT
  Cable3 : Lib_EMTAT/Components/Power Flow/Cable  R=0.2
      settings: SourceProductName=EMTAT
  Constant{,1,3..14} (14 alike) : Constant  Value=0
  Constant2 : Constant  Value=350
  Current Junction : Lib_EMTAT/Components/Power Flow/Current Junction  Nb=1
      settings: SourceProductName=EMTAT
      settings: AttributesFormatString=|
      | Current Junction
      | Version: %<LibraryVersion>
  DC-DC Converter : Lib_EMTAT/Components/Power Flow/DC-DC Converter (Set Output Voltage)  X_Vin_VoltageVec_M=[0 100 1000 5000]  Y_Iout_CurrentVec_M=[0 10 100 150]  T_C_PlossArray_M=0.98*ones(4,4)  FM=0  Plosslim=0
      settings: SourceProductName=EMTAT
  Display1 : Display
  Display9 : Display
  Integrator1 : Integrator  InitialCondition=150
  Integrator2 : Integrator  InitialCondition=2000
  Integrator3 : Integrator  InitialCondition=2000
  Inverter/Rectifier (Sink)1 : Lib_EMTAT/Components/Power Flow/DC-AC Inverter  X_C_VoltageInVec_M=[0 400]  Y_C_RMSCurrentOutVec_M=[0 300]  T_C_PowLossArray_M=[1000 1000;1000 1000]  K_e=0.0503  FM=0  Plosslim=0
      settings: SourceProductName=EMTAT
  Inverter/Rectifier (Sink)2 : Lib_EMTAT/Components/Power Flow/DC-AC Inverter  X_C_VoltageInVec_M=[0 400]  Y_C_RMSCurrentOutVec_M=[0 300]  T_C_PowLossArray_M=[1000 1000;1000 1000]  K_e=0.0503  FM=0  Plosslim=0
      settings: SourceProductName=EMTAT
  Mechanical Shaft1 : Lib_EMTAT/Components/Power Flow/Mechanical Shaft  J=0.01  B=0.001
      settings: SourceProductName=EMTAT
  Mechanical Shaft2 : Lib_EMTAT/Components/Power Flow/Mechanical Shaft  J=0.01  B=0.001
      settings: SourceProductName=EMTAT
  Motor/Generator (Sink)1 : Lib_EMTAT/Components/Power Flow/Three Phase Electric Machine (Sink)  X_C_SpeedVec_M=[0 100 1000 5000]  Y_C_TorqueVec_M=[0 10 100 150]  T_C_EffArray_M=0.99*ones(4,4)  FM=0
      settings: SourceProductName=EMTAT
  Motor/Generator (Sink)2 : Lib_EMTAT/Components/Power Flow/Three Phase Electric Machine (Sink)  X_C_SpeedVec_M=[0 100 1000 5000]  Y_C_TorqueVec_M=[0 10 100 150]  T_C_EffArray_M=0.99*ones(4,4)  FM=0
      settings: SourceProductName=EMTAT
  Mux : Mux  Inputs=2
  Mux1 : Mux  Inputs=2
  Sum of Elements : Sum  Inputs=+
  Super Capacitor : Lib_EMTAT/Components/Power Flow/Supercapacitor  C=130  ESR=0.02  TSE=0  BlkNm=double(gcb)
      settings: SourceProductName=EMTAT
  Terminator{1..13,17..19,21..24} (20 alike) : Terminator
  Unit Delay1 : UnitDelay  SampleTime=-1  HasFrameUpgradeWarning=on
  Unit Delay2 : UnitDelay  SampleTime=-1  HasFrameUpgradeWarning=on
  Unit Delay3 : UnitDelay  SampleTime=-1  HasFrameUpgradeWarning=on
  Vout : Outport
  Idmd : Outport  Port=2
  wires:
  Constant14/1 -> DC-DC Converter/5
  Constant13/1 -> DC-DC Converter/4
  Constant12/1 -> Cable3/3
  Mechanical Shaft2/2 -> Terminator24/1
  Mechanical Shaft2/1 -> Terminator1/1
  Constant11/1 -> Mechanical Shaft2/2
  Constant10/1 -> Mechanical Shaft1/2
  Mechanical Shaft1/3 -> Integrator2/1
  Motor/Generator (Sink)2/3 -> Terminator10/1
  Constant8/1 -> Inverter/Rectifier (Sink)2/4
  Inverter/Rectifier (Sink)2/1 -> Display1/1, Motor/Generator (Sink)2/1
  [N_M2] -> Motor/Generator (Sink)2/2
  Cable3/1 -> Inverter/Rectifier (Sink)2/1
  Motor/Generator (Sink)2/4 -> Inverter/Rectifier (Sink)2/3
  Constant6/1 -> Motor/Generator (Sink)2/4
  Inverter/Rectifier (Sink)2/4 -> Cable3/2
  [Tset_2] -> Motor/Generator (Sink)2/3
  Inverter/Rectifier (Sink)2/3 -> Terminator9/1
  [N_M2] -> Inverter/Rectifier (Sink)2/2
  Constant7/1 -> Motor/Generator (Sink)2/5
  Inverter/Rectifier (Sink)2/2 -> Terminator4/1
  Constant9/1 -> Inverter/Rectifier (Sink)2/5
  Constant5/1 -> Cable1/3
  Constant4/1 -> Inverter/Rectifier (Sink)1/5
  Constant3/1 -> Inverter/Rectifier (Sink)1/4
  Motor/Generator (Sink)1/3 -> Terminator7/1
  Constant1/1 -> Motor/Generator (Sink)1/5
  Constant/1 -> Motor/Generator (Sink)1/4
  Tset/1 -> Bus Selector1/1
  Bus Selector1/2 -> [Tset_2]  "<Tset 1-4-2>"
  Bus Selector1/1 -> [Tset_1]  "<Tset 1-4-1>"
  Sum of Elements/1 -> Idmd/1, Mux/2
  Mux1/1 -> Sum of Elements/1
  Motor/Generator (Sink)1/1 -> Mechanical Shaft1/1
  Inverter/Rectifier (Sink)1/2 -> Terminator5/1
  DC-DC Converter/3 -> Terminator23/1
  DC-DC Converter/2 -> Terminator22/1
  Mechanical Shaft1/1 -> Terminator17/1
  Motor/Generator (Sink)2/2 -> Terminator21/1
  Super Capacitor/3 -> Terminator12/1
  Cable1/2 -> Terminator18/1
  Motor/Generator (Sink)2/1 -> Mechanical Shaft2/1
  Cable3/3 -> Terminator3/1
  Motor/Generator (Sink)1/2 -> Terminator8/1
  Constant2/1 -> DC-DC Converter/1
  Cable1/4 -> Mux1/1
  Unit Delay1/1 -> Super Capacitor/3
  Super Capacitor/5 -> Unit Delay1/1
  Inverter/Rectifier (Sink)1/3 -> Terminator6/1
  Cable1/5 -> Unit Delay2/1
  Integrator1/1 -> Super Capacitor/2
  Inverter/Rectifier (Sink)1/4 -> Cable1/2
  Unit Delay3/1 -> Cable3/4
  Cable1/3 -> Terminator19/1
  Integrator3/1 -> Mechanical Shaft2/3, [N_M2]
  Cable3/4 -> Mux1/2
  Super Capacitor/2 -> Terminator11/1
  Inverter/Rectifier (Sink)1/1 -> Display9/1, Motor/Generator (Sink)1/1
  Cable3/5 -> Unit Delay3/1
  [N_M1] -> Inverter/Rectifier (Sink)1/2
  Cable1/1 -> Inverter/Rectifier (Sink)1/1
  Integrator2/1 -> Mechanical Shaft1/3, [N_M1]
  Mux/1 -> Current Junction/1
  Current Junction/1 -> DC-DC Converter/3
  DC-DC Converter/4 -> Super Capacitor/1
  Cable3/2 -> Terminator2/1
  Unit Delay2/1 -> Cable1/4
  Mechanical Shaft1/2 -> Terminator13/1
  [N_M1] -> Motor/Generator (Sink)1/2
  Super Capacitor/1 -> DC-DC Converter/2
  Super Capacitor/4 -> Integrator1/1
  Motor/Generator (Sink)1/4 -> Inverter/Rectifier (Sink)1/3
  DC-DC Converter/1 -> Cable1/1, Vout/1, Cable3/1
  [Tset_1] -> Motor/Generator (Sink)1/3
  Mechanical Shaft2/3 -> Integrator3/1
  Iin/1 -> Mux/1
